simulink model "RGB_Color_Component_ManualThreshold"  (R2016a)
settings: Solver=VariableStepAuto  StartTime=0.0  StopTime=10.0  RelTol=1e-3
undefined symbols (not defined in the file): Rec, SDTV
libraries: visionconversions x2, visionsources x1, visionsinks x1
settings Model: Creator=YASARA  LastModifiedBy=YASARA

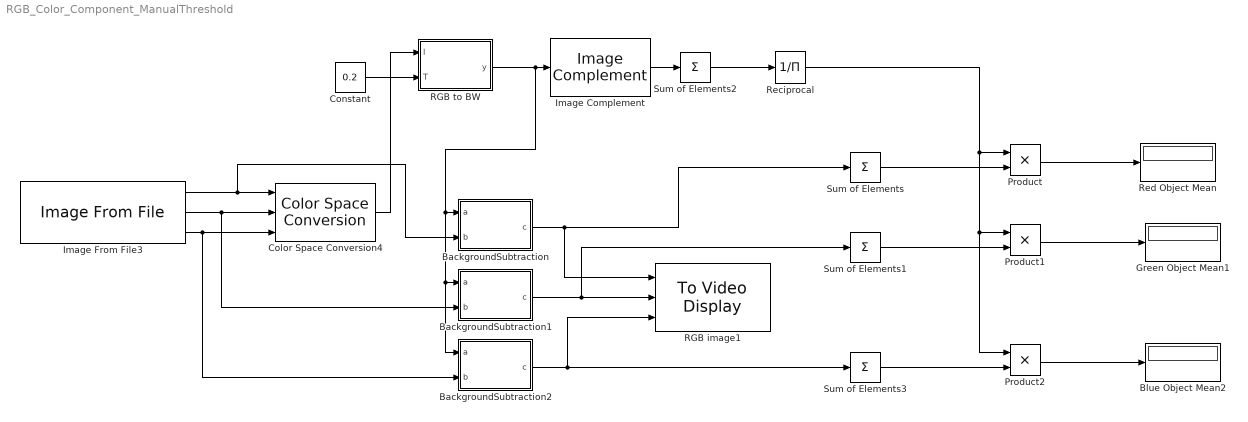
== system RGB_Color_Component_ManualThreshold ==
  BackgroundSubtraction : MATLAB Function  TreatAsAtomicUnit=on
  BackgroundSubtraction1 : MATLAB Function  TreatAsAtomicUnit=on
  BackgroundSubtraction2 : MATLAB Function  TreatAsAtomicUnit=on
  Blue Object Mean2 : Display
  Color Space Conversion4 : visionconversions/Color Space  Conversion  conversion=Obsolete  conversionActive=R'G'B' to intensity  wp_str=D65  rec=Rec. 601 (SDTV)  sys=1125/60/2:1  imagePorts=Separate color signals
  Constant : Constant  Value=0.2  SampleTime=1
  Green Object Mean1 : Display
  Image Complement : visionconversions/Image Complement
  Image From File3 : visionsources/Image From File  Tag=vipblks_nd  FileName=C:\Users\YASARA\Desktop\sampl\G200B200R200.jpg  imagePorts=Separate color signals  Ts=1  ImageDataType=uint8  Signed=on  WordLength=16  sdImageDataType=uint(8)  FractionLengthMode=User-defined  FractionLength=15  OutPortLabels=R|G|B
  Product : Product
  Product1 : Product
  Product2 : Product
  RGB image1 : visionsinks/To Video Display  windowSizeMode=Normal  openAtMdlStart=on  fullScreen=off  videoWindowX=70  videoWindowY=162  saveWindowSize=off  videoWindowWidth=512  videoWindowHeight=384  inputColorFormat=RGB  inputType=Obsolete  imagePorts=Separate color signals  OutputDevice=On-screen video monitor  dataOrg=Column-major  isWindowOpen=off
  RGB to BW : MATLAB Function  TreatAsAtomicUnit=on
  Reciprocal : Product  Inputs=/  OutDataTypeStr=double  SaturateOnIntegerOverflow=on  RndMeth=Zero
  Red Object Mean : Display
  Sum of Elements : Sum  Inputs=+
  Sum of Elements1 : Sum  Inputs=+
  Sum of Elements2 : Sum  Inputs=+  AccumDataTypeStr=double  OutDataTypeStr=double  RndMeth=Nearest
  Sum of Elements3 : Sum  Inputs=+
  wires:
  Color Space Conversion4/1 -> RGB to BW/1(I)
  Sum of Elements/1 -> Product/2
  BackgroundSubtraction/1(c) -> RGB image1/1, Sum of Elements/1
  BackgroundSubtraction1/1(c) -> RGB image1/2, Sum of Elements1/1
  Sum of Elements3/1 -> Product2/2
  BackgroundSubtraction2/1(c) -> RGB image1/3, Sum of Elements3/1
  Constant/1 -> RGB to BW/2(T)
  Sum of Elements2/1 -> Reciprocal/1
  Product/1 -> Red Object Mean/1
  Sum of Elements1/1 -> Product1/2
  Product1/1 -> Green Object Mean1/1
  Product2/1 -> Blue Object Mean2/1
  Reciprocal/1 -> Product/1, Product1/1, Product2/1
  RGB to BW/1(y) -> Image Complement/1, BackgroundSubtraction2/1(a), BackgroundSubtraction1/1(a), BackgroundSubtraction/1(a)
  Image From File3/1 -> BackgroundSubtraction/2(b), Color Space Conversion4/1
  Image From File3/2 -> BackgroundSubtraction1/2(b), Color Space Conversion4/2
  Image From File3/3 -> BackgroundSubtraction2/2(b), Color Space Conversion4/3
  Image Complement/1 -> Sum of Elements2/1

== matlab function RGB_Color_Component_ManualThreshold/BackgroundSubtraction1 ==
  data: a input; b input; c output
function c = fcn(a,b)
%#codegen
c=double(uint8(a).*b);
return

== matlab function RGB_Color_Component_ManualThreshold/RGB to BW ==
  data: I input; y output; T input
function y = fcn(I,T)
%#codegen
BW = imbinarize(I,T);
y = BW;

== matlab function RGB_Color_Component_ManualThreshold/BackgroundSubtraction2 ==
  data: a input; b input; c output
function c = fcn(a,b)
%#codegen
c=double(uint8(a).*b);
return

== matlab function RGB_Color_Component_ManualThreshold/BackgroundSubtraction ==
  data: a input; b input; c output
function c = fcn(a,b)
%#codegen
c=double(uint8(a).*b);
return
